simulink model "PIDTu4_1920"  (Simulink 5.0)
settings: Solver=ode45  StartTime=0.0  StopTime=5  RelTol=1e-3
libraries: simulink_extras x3
settings Model: LastModifiedBy=ThinkPad

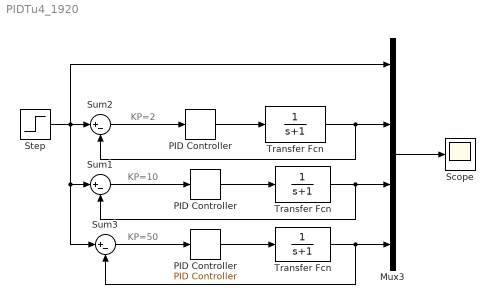
== system PIDTu4_1920 ==
  note: KP=2
  note: KP=10
  note: KP=50
  " PID Controller " : simulink_extras/Additional Linear/PID Controller  P=20  I=0  D=0
  " Transfer Fcn " : TransferFcn  Denominator=[1 1]
  Mux3 : Mux
  PID Controller : simulink_extras/Additional Linear/PID Controller  P=2  I=0  D=0
  "PID Controller " : simulink_extras/Additional Linear/PID Controller  P=10  I=0  D=0
  Scope : Scope
      settings: TimeRange=1.6  YMin=0.5  YMax=1  SaveName=PIDtu4_20  DataFormat=Array  MaxDataPoints=500000
  Step : Step  Time=0  SampleTime=0
  Sum1 : Sum  Inputs=|+-  SaturateOnIntegerOverflow=on
  Sum2 : Sum  Inputs=|+-  SaturateOnIntegerOverflow=on
  Sum3 : Sum  Inputs=|+-  SaturateOnIntegerOverflow=on
  Transfer Fcn : TransferFcn  Denominator=[1 1]
  "Transfer Fcn " : TransferFcn  Denominator=[1 1]
  wires:
  Step/1 -> Sum2/1, Mux3/1, Sum1/1, Sum3/1
  Sum2/1 -> PID Controller/1
  PID Controller/1 -> Transfer Fcn/1
  Transfer Fcn/1 -> Mux3/2, Sum2/2
  Sum1/1 -> "PID Controller "/1
  "PID Controller "/1 -> " Transfer Fcn "/1
  Sum3/1 -> " PID Controller "/1
  " PID Controller "/1 -> "Transfer Fcn "/1
  " Transfer Fcn "/1 -> Mux3/3, Sum1/2
  "Transfer Fcn "/1 -> Mux3/4, Sum3/2
  Mux3/1 -> Scope/1
